simulink model "TestModeleBatteries"  (R2019b)
settings: Solver=VariableStepAuto  StartTime=0.0  StopTime=10.0  RelTol=1e-3
values from neighbouring files (symbols this model uses):
  ess_coulombic_eff = 0.99    [Batteries.m]
  ess_max_ah_cap = 28    [Batteries.m]
  ess_module_number = 20    [Batteries.m]
  ess_r = [0.01266 0.00685	0.00644	0.00599	0.00587	0.00575	0.00568	0.00581	0.00623	0.00667  0.00635]    [Batteries.m]
  ess_soc = [0:.1:1]    [Batteries.m]
  ess_tau = 0.1    [Batteries.m]
  ess_voc = [12.5 12.8 13.1 13.3 13.4 13.4 13.5 13.6 13.7 13.9 14.2]    [Batteries.m]
  SocInit = 0.8    [Batteries.m]
settings Model: Creator=szhang6_  LastModifiedBy=szhang6_
settings DataIOCC: ReturnWorkspaceOutputs=off

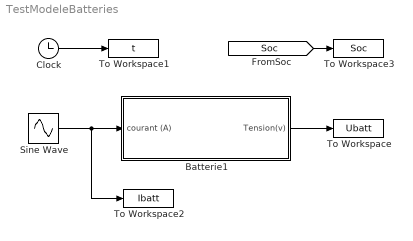
== system TestModeleBatteries ==
  Batterie1 : Subsystem
  Clock : Clock
  Sine Wave : Sin  Amplitude=100  Frequency=0.5*2*pi  SampleTime=0
  To Workspace : ToWorkspace  VariableName=Ubatt  SampleTime=-1
  To Workspace1 : ToWorkspace  VariableName=t  SampleTime=-1
  To Workspace2 : ToWorkspace  VariableName=Ibatt  SampleTime=-1
  To Workspace3 : ToWorkspace  VariableName=Soc  SampleTime=-1
  wires:
  Clock/1 -> To Workspace1/1
  [Soc] -> To Workspace3/1
  Sine Wave/1 -> To Workspace2/1, Batterie1/1(courant (A))
  Batterie1/1(Tension(v)) -> To Workspace/1

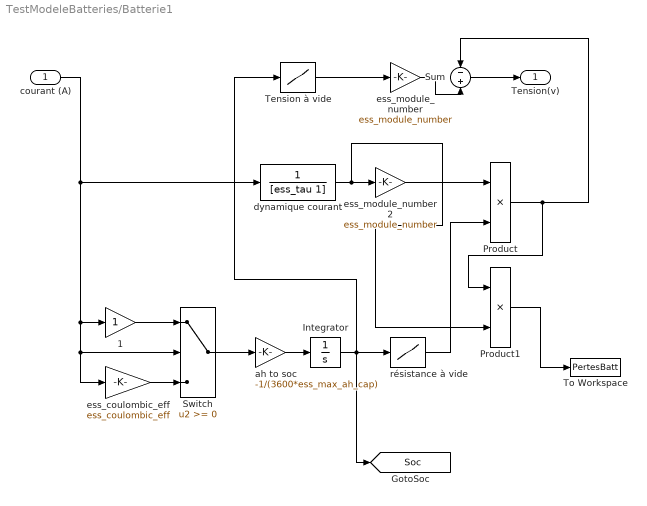
== system TestModeleBatteries/Batterie1 ==
  courant (A) : Inport
  1 : Gain
  Integrator : Integrator  InitialCondition=SocInit
  Product : Product  Inputs=**
  Product1 : Product  Inputs=**
  Sum : Sum  Inputs=-+
  Switch : Switch
  Tension à vide : Lookup  InputValues=ess_soc  Table=ess_voc
  To Workspace : ToWorkspace  VariableName=PertesBatt  SampleTime=-1
  "ah to soc " : Gain  Gain=-1/(3600*ess_max_ah_cap)
  dynamique courant : TransferFcn  Denominator=[ess_tau 1]
  "ess_coulombic_eff " : Gain  Gain=ess_coulombic_eff
  "ess_module_number " : Gain  Gain=ess_module_number
  ess_module_number 2 : Gain  Gain=ess_module_number
  résistance à vide : Lookup  InputValues=ess_soc  Table=ess_r
  Tension(v) : Outport
  tag scope: Soc=global
  wires:
  courant (A)/1 -> dynamique courant/1, "ess_coulombic_eff "/1, Switch/2, 1/1
  1/1 -> Switch/1
  "ess_coulombic_eff "/1 -> Switch/3
  Switch/1 -> "ah to soc "/1
  "ah to soc "/1 -> Integrator/1
  dynamique courant/1 -> Product1/2, ess_module_number 2/1
  Integrator/1 -> Tension à vide/1, résistance à vide/1, [Soc]
  ess_module_number 2/1 -> Product/1
  résistance à vide/1 -> Product/2
  Product/1 -> Product1/1, Sum/1
  Sum/1 -> Tension(v)/1
  Tension à vide/1 -> "ess_module_number "/1
  "ess_module_number "/1 -> Sum/2
  Product1/1 -> To Workspace/1
